simulink model "siciliano_position"  (R2020b)
settings: Solver=ode4  StartTime=0.0  StopTime=10  FixedStep=1e-5  MaxStep=1e-4  RelTol=1e-4  EnableMultiTasking=on
values from neighbouring files (symbols this model uses):
  D = 0.9    [siciliano_position_params.m]
  dm = 0.0068    [siciliano_position_params.m]
  Jm = 0.0104    [siciliano_position_params.m]
  P = 10    [siciliano_position_params.m]
  Ra = 0.68    [siciliano_position_params.m]
undefined symbols (not defined in the file or in its folder): kt, kv
settings Model: Creator=eldisondimo  LastModifiedBy=filippo
settings DataIOCC: LimitDataPoints=on  SaveOutput=off  SaveTime=off  ReturnWorkspaceOutputs=off
settings OptimizationCC: ExpressionDepthLimit=2147483647  LifeSpan=1
settings DebuggingCC: UnderspecifiedInitializationDetection=Classic  MergeDetectMultiDrivingBlocksExec=none  FcnCallInpInsideContextMsg=warning  AllowSymbolicDim=off  StateNameClashWarn=warning  SFUnexpectedBacktrackingDiag=warning  SFNoUnconditionalDefaultTransitionDiag=warning  SFExecutionAtInitializationDiag=none  ArithmeticOperatorsInVariantConditions=warning
settings SFSimCC: SimUseLocalCustomCode=off  CustomCodeUndefinedFunction=UseInterfaceOnly
settings RTWCC: RTWUseLocalCustomCode=off
settings CodeAppCC: StateflowObjectComments=on
settings GRTTargetCC: TargetLangStandard=C89/C90 (ANSI)  CombineOutputUpdateFcns=off  GRTInterface=on

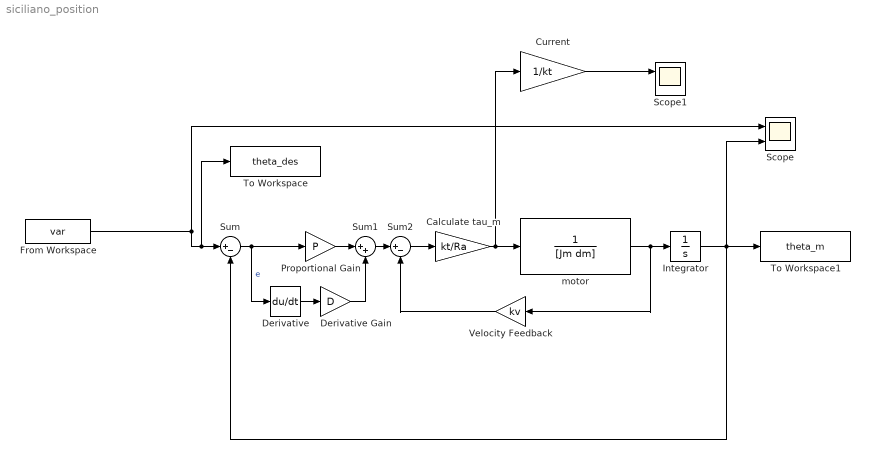
== system siciliano_position ==
  Calculate tau_m : Gain  Gain=kt/Ra
  Current : Gain  Gain=1/kt
  Derivative : Derivative
  Derivative Gain : Gain  Gain=D
  From Workspace : FromWorkspace  VariableName=var
  Integrator : Integrator
  Proportional Gain : Gain  Gain=P
  Scope : Scope  NumInputPorts=2
  Scope1 : Scope  NumInputPorts=2
  Sum : Sum  Inputs=|+-
  Sum1 : Sum  Inputs=|++
  Sum2 : Sum  Inputs=|+-
  To Workspace : ToWorkspace  VariableName=theta_des  SaveFormat=Structure With Time  SampleTime=-1
  To Workspace1 : ToWorkspace  VariableName=theta_m  SaveFormat=Structure With Time  SampleTime=-1
  Velocity Feedback : Gain  Gain=kv
  "motor " : TransferFcn  Denominator=[Jm dm]
  wires:
  Sum/1 -> Proportional Gain/1, Derivative/1  "e"
  From Workspace/1 -> Scope/1, To Workspace/1, Sum/1
  "motor "/1 -> Velocity Feedback/1, Integrator/1
  Proportional Gain/1 -> Sum1/1
  Derivative Gain/1 -> Sum1/2
  Derivative/1 -> Derivative Gain/1
  Integrator/1 -> Scope/2, To Workspace1/1, Sum/2
  Calculate tau_m/1 -> Current/1, "motor "/1
  Sum1/1 -> Sum2/1
  Sum2/1 -> Calculate tau_m/1
  Velocity Feedback/1 -> Sum2/2
  Current/1 -> Scope1/1
